simulink model "RxCAN2"  (R2014a)
settings: Solver=ode45  StartTime=0.0  StopTime=10.0  RelTol=1e-3
libraries: simulink x16
settings Model: Creator=10226  LastModifiedBy=10226

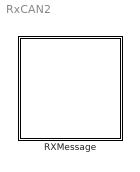
== system RxCAN2 ==
  RXMessage : Subsystem

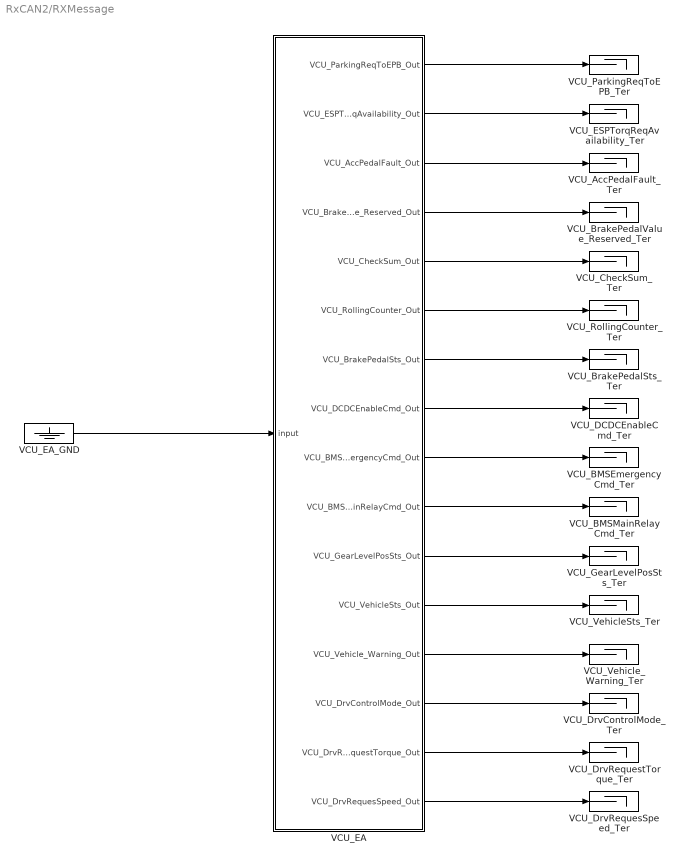
== system RxCAN2/RXMessage ==
  VCU_AccPedalFault_Ter : Terminator
  VCU_BMSEmergencyCmd_Ter : Terminator
  VCU_BMSMainRelayCmd_Ter : Terminator
  VCU_BrakePedalSts_Ter : Terminator
  VCU_BrakePedalValue_Reserved_Ter : Terminator
  VCU_CheckSum_Ter : Terminator
  VCU_DCDCEnableCmd_Ter : Terminator
  VCU_DrvControlMode_Ter : Terminator
  VCU_DrvRequesSpeed_Ter : Terminator
  VCU_DrvRequestTorque_Ter : Terminator
  VCU_EA : Subsystem
  VCU_EA_GND : Ground
  VCU_ESPTorqReqAvailability_Ter : Terminator
  VCU_GearLevelPosSts_Ter : Terminator
  VCU_ParkingReqToEPB_Ter : Terminator
  VCU_RollingCounter_Ter : Terminator
  VCU_VehicleSts_Ter : Terminator
  VCU_Vehicle_Warning_Ter : Terminator
  wires:
  VCU_EA/1(VCU_ParkingReqToEPB_Out) -> VCU_ParkingReqToEPB_Ter/1
  VCU_EA/2(VCU_ESPTorqReqAvailability_Out) -> VCU_ESPTorqReqAvailability_Ter/1
  VCU_EA/3(VCU_AccPedalFault_Out) -> VCU_AccPedalFault_Ter/1
  VCU_EA/4(VCU_BrakePedalValue_Reserved_Out) -> VCU_BrakePedalValue_Reserved_Ter/1
  VCU_EA/5(VCU_CheckSum_Out) -> VCU_CheckSum_Ter/1
  VCU_EA/6(VCU_RollingCounter_Out) -> VCU_RollingCounter_Ter/1
  VCU_EA/7(VCU_BrakePedalSts_Out) -> VCU_BrakePedalSts_Ter/1
  VCU_EA/8(VCU_DCDCEnableCmd_Out) -> VCU_DCDCEnableCmd_Ter/1
  VCU_EA/9(VCU_BMSEmergencyCmd_Out) -> VCU_BMSEmergencyCmd_Ter/1
  VCU_EA/10(VCU_BMSMainRelayCmd_Out) -> VCU_BMSMainRelayCmd_Ter/1
  VCU_EA/11(VCU_GearLevelPosSts_Out) -> VCU_GearLevelPosSts_Ter/1
  VCU_EA/12(VCU_VehicleSts_Out) -> VCU_VehicleSts_Ter/1
  VCU_EA/13(VCU_Vehicle_Warning_Out) -> VCU_Vehicle_Warning_Ter/1
  VCU_EA/14(VCU_DrvControlMode_Out) -> VCU_DrvControlMode_Ter/1
  VCU_EA/15(VCU_DrvRequestTorque_Out) -> VCU_DrvRequestTorque_Ter/1
  VCU_EA/16(VCU_DrvRequesSpeed_Out) -> VCU_DrvRequesSpeed_Ter/1
  VCU_EA_GND/1 -> VCU_EA/1(input)

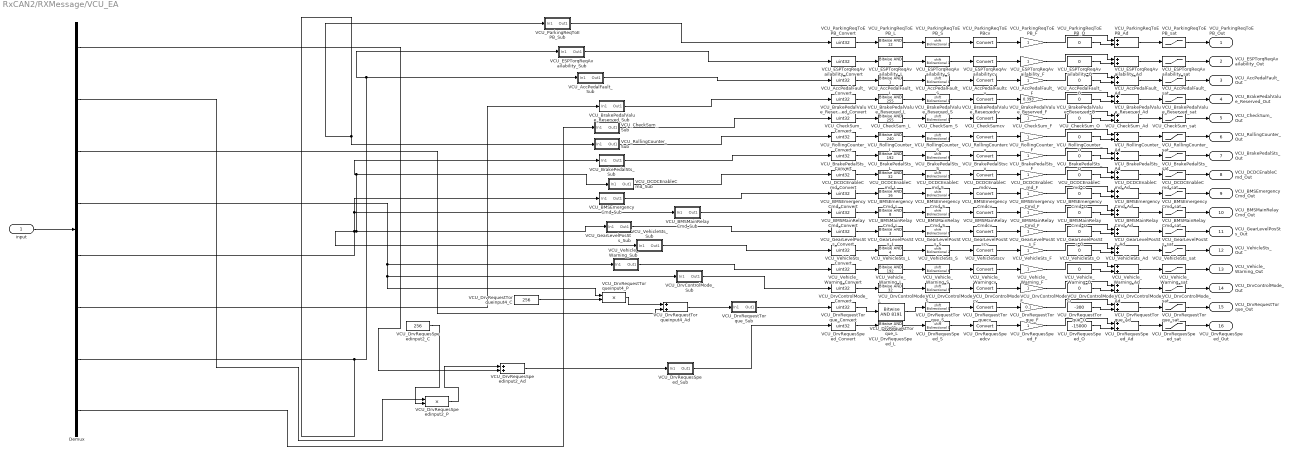
== system RxCAN2/RXMessage/VCU_EA ==
  input : Inport
  Demux : Demux  Outputs=8
  VCU_AccPedalFault_Ad : Sum
  VCU_AccPedalFault_Convert : DataTypeConversion  OutDataTypeStr=uint32
  VCU_AccPedalFault_F : Gain
  VCU_AccPedalFault_L : simulink/Logic and Bit Operations/Bitwise Operator  logicop=AND  UseBitMask=on  BitMask=1  BitMaskRealWorld=Stored Integer
  VCU_AccPedalFault_O : Constant  Value=0  OutDataTypeStr=single
  VCU_AccPedalFault_S : ArithShift
  VCU_AccPedalFault_Sub : Subsystem
  VCU_AccPedalFault_sat : Saturate  UpperLimit=1  LowerLimit=0
  VCU_AccPedalFaultcv : DataTypeConversion
  VCU_BMSEmergencyCmd_Ad : Sum
  VCU_BMSEmergencyCmd_Convert : DataTypeConversion  OutDataTypeStr=uint32
  VCU_BMSEmergencyCmd_F : Gain
  VCU_BMSEmergencyCmd_L : simulink/Logic and Bit Operations/Bitwise Operator  logicop=AND  UseBitMask=on  BitMask=16  BitMaskRealWorld=Stored Integer
  VCU_BMSEmergencyCmd_O : Constant  Value=0  OutDataTypeStr=single
  VCU_BMSEmergencyCmd_S : ArithShift  BitShiftNumber=4
  VCU_BMSEmergencyCmd_Sub : Subsystem
  VCU_BMSEmergencyCmd_sat : Saturate  UpperLimit=1  LowerLimit=0
  VCU_BMSEmergencyCmdcv : DataTypeConversion
  VCU_BMSMainRelayCmd_Ad : Sum
  VCU_BMSMainRelayCmd_Convert : DataTypeConversion  OutDataTypeStr=uint32
  VCU_BMSMainRelayCmd_F : Gain
  VCU_BMSMainRelayCmd_L : simulink/Logic and Bit Operations/Bitwise Operator  logicop=AND  UseBitMask=on  BitMask=8  BitMaskRealWorld=Stored Integer
  VCU_BMSMainRelayCmd_O : Constant  Value=0  OutDataTypeStr=single
  VCU_BMSMainRelayCmd_S : ArithShift  BitShiftNumber=3
  VCU_BMSMainRelayCmd_Sub : Subsystem
  VCU_BMSMainRelayCmd_sat : Saturate  UpperLimit=1  LowerLimit=0
  VCU_BMSMainRelayCmdcv : DataTypeConversion
  VCU_BrakePedalSts_Ad : Sum
  VCU_BrakePedalSts_Convert : DataTypeConversion  OutDataTypeStr=uint32
  VCU_BrakePedalSts_F : Gain
  VCU_BrakePedalSts_L : simulink/Logic and Bit Operations/Bitwise Operator  logicop=AND  UseBitMask=on  BitMask=192  BitMaskRealWorld=Stored Integer
  VCU_BrakePedalSts_O : Constant  Value=0  OutDataTypeStr=single
  VCU_BrakePedalSts_S : ArithShift  BitShiftNumber=6
  VCU_BrakePedalSts_Sub : Subsystem
  VCU_BrakePedalSts_sat : Saturate  UpperLimit=3  LowerLimit=0
  VCU_BrakePedalStscv : DataTypeConversion
  VCU_BrakePedalValue_Reserved_Ad : Sum
  VCU_BrakePedalValue_Reserved_Convert : DataTypeConversion  OutDataTypeStr=uint32
  VCU_BrakePedalValue_Reserved_F : Gain  Gain=0.393
  VCU_BrakePedalValue_Reserved_L : simulink/Logic and Bit Operations/Bitwise Operator  logicop=AND  UseBitMask=on  BitMask=255  BitMaskRealWorld=Stored Integer
  VCU_BrakePedalValue_Reserved_O : Constant  Value=0  OutDataTypeStr=single
  VCU_BrakePedalValue_Reserved_S : ArithShift
  VCU_BrakePedalValue_Reserved_Sub : Subsystem
  VCU_BrakePedalValue_Reserved_sat : Saturate  UpperLimit=100  LowerLimit=0
  VCU_BrakePedalValue_Reservedcv : DataTypeConversion
  VCU_CheckSum_Ad : Sum
  VCU_CheckSum_Convert : DataTypeConversion  OutDataTypeStr=uint32
  VCU_CheckSum_F : Gain
  VCU_CheckSum_L : simulink/Logic and Bit Operations/Bitwise Operator  logicop=AND  UseBitMask=on  BitMask=255  BitMaskRealWorld=Stored Integer
  VCU_CheckSum_O : Constant  Value=0  OutDataTypeStr=single
  VCU_CheckSum_S : ArithShift
  VCU_CheckSum_Sub : Subsystem
  VCU_CheckSum_sat : Saturate  UpperLimit=255  LowerLimit=0
  VCU_CheckSumcv : DataTypeConversion
  VCU_DCDCEnableCmd_Ad : Sum
  VCU_DCDCEnableCmd_Convert : DataTypeConversion  OutDataTypeStr=uint32
  VCU_DCDCEnableCmd_F : Gain
  VCU_DCDCEnableCmd_L : simulink/Logic and Bit Operations/Bitwise Operator  logicop=AND  UseBitMask=on  BitMask=32  BitMaskRealWorld=Stored Integer
  VCU_DCDCEnableCmd_O : Constant  Value=0  OutDataTypeStr=single
  VCU_DCDCEnableCmd_S : ArithShift  BitShiftNumber=5
  VCU_DCDCEnableCmd_Sub : Subsystem
  VCU_DCDCEnableCmd_sat : Saturate  UpperLimit=1  LowerLimit=0
  VCU_DCDCEnableCmdcv : DataTypeConversion
  VCU_DrvControlMode_Ad : Sum
  VCU_DrvControlMode_Convert : DataTypeConversion  OutDataTypeStr=uint32
  VCU_DrvControlMode_F : Gain
  VCU_DrvControlMode_L : simulink/Logic and Bit Operations/Bitwise Operator  logicop=AND  UseBitMask=on  BitMask=32  BitMaskRealWorld=Stored Integer
  VCU_DrvControlMode_O : Constant  Value=0  OutDataTypeStr=single
  VCU_DrvControlMode_S : ArithShift  BitShiftNumber=5
  VCU_DrvControlMode_Sub : Subsystem
  VCU_DrvControlMode_sat : Saturate  UpperLimit=1  LowerLimit=0
  VCU_DrvControlModecv : DataTypeConversion
  VCU_DrvRequesSpeed_Ad : Sum
  VCU_DrvRequesSpeed_Convert : DataTypeConversion  OutDataTypeStr=uint32
  VCU_DrvRequesSpeed_F : Gain
  VCU_DrvRequesSpeed_L : simulink/Logic and Bit Operations/Bitwise Operator  logicop=AND  UseBitMask=on  BitMask=65535  BitMaskRealWorld=Stored Integer
  VCU_DrvRequesSpeed_O : Constant  Value=-15000  OutDataTypeStr=single
  VCU_DrvRequesSpeed_S : ArithShift
  VCU_DrvRequesSpeed_Sub : Subsystem
  VCU_DrvRequesSpeed_sat : Saturate  UpperLimit=15000  LowerLimit=-15000
  VCU_DrvRequesSpeedcv : DataTypeConversion
  VCU_DrvRequesSpeedinput2_Ad : Sum
  VCU_DrvRequesSpeedinput2_C : Constant  Value=256
  VCU_DrvRequesSpeedinput2_P : Product
  VCU_DrvRequestTorque_Ad : Sum
  VCU_DrvRequestTorque_Convert : DataTypeConversion  OutDataTypeStr=uint32
  VCU_DrvRequestTorque_F : Gain  Gain=0.1
  VCU_DrvRequestTorque_L : simulink/Logic and Bit Operations/Bitwise Operator  logicop=AND  UseBitMask=on  BitMask=8191  BitMaskRealWorld=Stored Integer
  VCU_DrvRequestTorque_O : Constant  Value=-300  OutDataTypeStr=single
  VCU_DrvRequestTorque_S : ArithShift
  VCU_DrvRequestTorque_Sub : Subsystem
  VCU_DrvRequestTorque_sat : Saturate  UpperLimit=300  LowerLimit=-300
  VCU_DrvRequestTorquecv : DataTypeConversion
  VCU_DrvRequestTorqueinput4_Ad : Sum
  VCU_DrvRequestTorqueinput4_C : Constant  Value=256
  VCU_DrvRequestTorqueinput4_P : Product
  VCU_ESPTorqReqAvailability_Ad : Sum
  VCU_ESPTorqReqAvailability_Convert : DataTypeConversion  OutDataTypeStr=uint32
  VCU_ESPTorqReqAvailability_F : Gain
  VCU_ESPTorqReqAvailability_L : simulink/Logic and Bit Operations/Bitwise Operator  logicop=AND  UseBitMask=on  BitMask=2  BitMaskRealWorld=Stored Integer
  VCU_ESPTorqReqAvailability_O : Constant  Value=0  OutDataTypeStr=single
  VCU_ESPTorqReqAvailability_S : ArithShift  BitShiftNumber=1
  VCU_ESPTorqReqAvailability_Sub : Subsystem
  VCU_ESPTorqReqAvailability_sat : Saturate  UpperLimit=1  LowerLimit=0
  VCU_ESPTorqReqAvailabilitycv : DataTypeConversion
  VCU_GearLevelPosSts_Ad : Sum
  VCU_GearLevelPosSts_Convert : DataTypeConversion  OutDataTypeStr=uint32
  VCU_GearLevelPosSts_F : Gain
  VCU_GearLevelPosSts_L : simulink/Logic and Bit Operations/Bitwise Operator  logicop=AND  UseBitMask=on  BitMask=3  BitMaskRealWorld=Stored Integer
  VCU_GearLevelPosSts_O : Constant  Value=0  OutDataTypeStr=single
  VCU_GearLevelPosSts_S : ArithShift
  VCU_GearLevelPosSts_Sub : Subsystem
  VCU_GearLevelPosSts_sat : Saturate  UpperLimit=3  LowerLimit=0
  VCU_GearLevelPosStscv : DataTypeConversion
  VCU_ParkingReqToEPB_Ad : Sum
  VCU_ParkingReqToEPB_Convert : DataTypeConversion  OutDataTypeStr=uint32
  VCU_ParkingReqToEPB_F : Gain
  VCU_ParkingReqToEPB_L : simulink/Logic and Bit Operations/Bitwise Operator  logicop=AND  UseBitMask=on  BitMask=12  BitMaskRealWorld=Stored Integer
  VCU_ParkingReqToEPB_O : Constant  Value=0  OutDataTypeStr=single
  VCU_ParkingReqToEPB_S : ArithShift  BitShiftNumber=2
  VCU_ParkingReqToEPB_Sub : Subsystem
  VCU_ParkingReqToEPB_sat : Saturate  UpperLimit=3  LowerLimit=0
  VCU_ParkingReqToEPBcv : DataTypeConversion
  VCU_RollingCounter_Ad : Sum
  VCU_RollingCounter_Convert : DataTypeConversion  OutDataTypeStr=uint32
  VCU_RollingCounter_F : Gain
  VCU_RollingCounter_L : simulink/Logic and Bit Operations/Bitwise Operator  logicop=AND  UseBitMask=on  BitMask=240  BitMaskRealWorld=Stored Integer
  VCU_RollingCounter_O : Constant  Value=0  OutDataTypeStr=single
  VCU_RollingCounter_S : ArithShift  BitShiftNumber=4
  VCU_RollingCounter_Sub : Subsystem
  VCU_RollingCounter_sat : Saturate  UpperLimit=15  LowerLimit=0
  VCU_RollingCountercv : DataTypeConversion
  VCU_VehicleSts_Ad : Sum
  VCU_VehicleSts_Convert : DataTypeConversion  OutDataTypeStr=uint32
  VCU_VehicleSts_F : Gain
  VCU_VehicleSts_L : simulink/Logic and Bit Operations/Bitwise Operator  logicop=AND  UseBitMask=on  BitMask=4  BitMaskRealWorld=Stored Integer
  VCU_VehicleSts_O : Constant  Value=0  OutDataTypeStr=single
  VCU_VehicleSts_S : ArithShift  BitShiftNumber=2
  VCU_VehicleSts_Sub : Subsystem
  VCU_VehicleSts_sat : Saturate  UpperLimit=1  LowerLimit=0
  VCU_VehicleStscv : DataTypeConversion
  VCU_Vehicle_Warning_Ad : Sum
  VCU_Vehicle_Warning_Convert : DataTypeConversion  OutDataTypeStr=uint32
  VCU_Vehicle_Warning_F : Gain
  VCU_Vehicle_Warning_L : simulink/Logic and Bit Operations/Bitwise Operator  logicop=AND  UseBitMask=on  BitMask=192  BitMaskRealWorld=Stored Integer
  VCU_Vehicle_Warning_O : Constant  Value=0  OutDataTypeStr=single
  VCU_Vehicle_Warning_S : ArithShift  BitShiftNumber=6
  VCU_Vehicle_Warning_Sub : Subsystem
  VCU_Vehicle_Warning_sat : Saturate  UpperLimit=3  LowerLimit=0
  VCU_Vehicle_Warningcv : DataTypeConversion
  VCU_ParkingReqToEPB_Out : Outport
  VCU_ESPTorqReqAvailability_Out : Outport  Port=2
  VCU_AccPedalFault_Out : Outport  Port=3
  VCU_BrakePedalValue_Reserved_Out : Outport  Port=4
  VCU_CheckSum_Out : Outport  Port=5
  VCU_RollingCounter_Out : Outport  Port=6
  VCU_BrakePedalSts_Out : Outport  Port=7
  VCU_DCDCEnableCmd_Out : Outport  Port=8
  VCU_BMSEmergencyCmd_Out : Outport  Port=9
  VCU_BMSMainRelayCmd_Out : Outport  Port=10
  VCU_GearLevelPosSts_Out : Outport  Port=11
  VCU_VehicleSts_Out : Outport  Port=12
  VCU_Vehicle_Warning_Out : Outport  Port=13
  VCU_DrvControlMode_Out : Outport  Port=14
  VCU_DrvRequestTorque_Out : Outport  Port=15
  VCU_DrvRequesSpeed_Out : Outport  Port=16
  wires:
  VCU_ParkingReqToEPB_F/1 -> VCU_ParkingReqToEPB_Ad/1
  VCU_ParkingReqToEPB_O/1 -> VCU_ParkingReqToEPB_Ad/2
  VCU_ParkingReqToEPB_Ad/1 -> VCU_ParkingReqToEPB_sat/1
  VCU_ParkingReqToEPB_sat/1 -> VCU_ParkingReqToEPB_Out/1
  Demux/7 -> VCU_ESPTorqReqAvailability_Sub/1(In1), VCU_AccPedalFault_Sub/1(In1), VCU_RollingCounter_Sub/1(In1), VCU_ParkingReqToEPB_Sub/1(In1)
  VCU_ParkingReqToEPB_Sub/1(Out1) -> VCU_ParkingReqToEPB_Convert/1
  VCU_ParkingReqToEPB_Convert/1 -> VCU_ParkingReqToEPB_L/1
  VCU_ParkingReqToEPB_L/1 -> VCU_ParkingReqToEPB_S/1
  VCU_ParkingReqToEPB_S/1 -> VCU_ParkingReqToEPBcv/1
  VCU_ParkingReqToEPBcv/1 -> VCU_ParkingReqToEPB_F/1
  VCU_ESPTorqReqAvailability_F/1 -> VCU_ESPTorqReqAvailability_Ad/1
  VCU_ESPTorqReqAvailability_O/1 -> VCU_ESPTorqReqAvailability_Ad/2
  VCU_ESPTorqReqAvailability_Ad/1 -> VCU_ESPTorqReqAvailability_sat/1
  VCU_ESPTorqReqAvailability_sat/1 -> VCU_ESPTorqReqAvailability_Out/1
  VCU_ESPTorqReqAvailability_Sub/1(Out1) -> VCU_ESPTorqReqAvailability_Convert/1
  VCU_ESPTorqReqAvailability_Convert/1 -> VCU_ESPTorqReqAvailability_L/1
  VCU_ESPTorqReqAvailability_L/1 -> VCU_ESPTorqReqAvailability_S/1
  VCU_ESPTorqReqAvailability_S/1 -> VCU_ESPTorqReqAvailabilitycv/1
  VCU_ESPTorqReqAvailabilitycv/1 -> VCU_ESPTorqReqAvailability_F/1
  VCU_AccPedalFault_F/1 -> VCU_AccPedalFault_Ad/1
  VCU_AccPedalFault_O/1 -> VCU_AccPedalFault_Ad/2
  VCU_AccPedalFault_Ad/1 -> VCU_AccPedalFault_sat/1
  VCU_AccPedalFault_sat/1 -> VCU_AccPedalFault_Out/1
  VCU_AccPedalFault_Sub/1(Out1) -> VCU_AccPedalFault_Convert/1
  VCU_AccPedalFault_Convert/1 -> VCU_AccPedalFault_L/1
  VCU_AccPedalFault_L/1 -> VCU_AccPedalFault_S/1
  VCU_AccPedalFault_S/1 -> VCU_AccPedalFaultcv/1
  VCU_AccPedalFaultcv/1 -> VCU_AccPedalFault_F/1
  VCU_BrakePedalValue_Reserved_F/1 -> VCU_BrakePedalValue_Reserved_Ad/1
  VCU_BrakePedalValue_Reserved_O/1 -> VCU_BrakePedalValue_Reserved_Ad/2
  VCU_BrakePedalValue_Reserved_Ad/1 -> VCU_BrakePedalValue_Reserved_sat/1
  VCU_BrakePedalValue_Reserved_sat/1 -> VCU_BrakePedalValue_Reserved_Out/1
  Demux/6 -> VCU_BrakePedalValue_Reserved_Sub/1(In1)
  VCU_BrakePedalValue_Reserved_Sub/1(Out1) -> VCU_BrakePedalValue_Reserved_Convert/1
  VCU_BrakePedalValue_Reserved_Convert/1 -> VCU_BrakePedalValue_Reserved_L/1
  VCU_BrakePedalValue_Reserved_L/1 -> VCU_BrakePedalValue_Reserved_S/1
  VCU_BrakePedalValue_Reserved_S/1 -> VCU_BrakePedalValue_Reservedcv/1
  VCU_BrakePedalValue_Reservedcv/1 -> VCU_BrakePedalValue_Reserved_F/1
  VCU_CheckSum_F/1 -> VCU_CheckSum_Ad/1
  VCU_CheckSum_O/1 -> VCU_CheckSum_Ad/2
  VCU_CheckSum_Ad/1 -> VCU_CheckSum_sat/1
  VCU_CheckSum_sat/1 -> VCU_CheckSum_Out/1
  Demux/8 -> VCU_CheckSum_Sub/1(In1)
  VCU_CheckSum_Sub/1(Out1) -> VCU_CheckSum_Convert/1
  VCU_CheckSum_Convert/1 -> VCU_CheckSum_L/1
  VCU_CheckSum_L/1 -> VCU_CheckSum_S/1
  VCU_CheckSum_S/1 -> VCU_CheckSumcv/1
  VCU_CheckSumcv/1 -> VCU_CheckSum_F/1
  VCU_RollingCounter_F/1 -> VCU_RollingCounter_Ad/1
  VCU_RollingCounter_O/1 -> VCU_RollingCounter_Ad/2
  VCU_RollingCounter_Ad/1 -> VCU_RollingCounter_sat/1
  VCU_RollingCounter_sat/1 -> VCU_RollingCounter_Out/1
  VCU_RollingCounter_Sub/1(Out1) -> VCU_RollingCounter_Convert/1
  VCU_RollingCounter_Convert/1 -> VCU_RollingCounter_L/1
  VCU_RollingCounter_L/1 -> VCU_RollingCounter_S/1
  VCU_RollingCounter_S/1 -> VCU_RollingCountercv/1
  VCU_RollingCountercv/1 -> VCU_RollingCounter_F/1
  VCU_BrakePedalSts_F/1 -> VCU_BrakePedalSts_Ad/1
  VCU_BrakePedalSts_O/1 -> VCU_BrakePedalSts_Ad/2
  VCU_BrakePedalSts_Ad/1 -> VCU_BrakePedalSts_sat/1
  VCU_BrakePedalSts_sat/1 -> VCU_BrakePedalSts_Out/1
  Demux/5 -> VCU_GearLevelPosSts_Sub/1(In1), VCU_BrakePedalSts_Sub/1(In1), VCU_DCDCEnableCmd_Sub/1(In1), VCU_VehicleSts_Sub/1(In1), VCU_BMSEmergencyCmd_Sub/1(In1), VCU_BMSMainRelayCmd_Sub/1(In1)
  VCU_BrakePedalSts_Sub/1(Out1) -> VCU_BrakePedalSts_Convert/1
  VCU_BrakePedalSts_Convert/1 -> VCU_BrakePedalSts_L/1
  VCU_BrakePedalSts_L/1 -> VCU_BrakePedalSts_S/1
  VCU_BrakePedalSts_S/1 -> VCU_BrakePedalStscv/1
  VCU_BrakePedalStscv/1 -> VCU_BrakePedalSts_F/1
  VCU_DCDCEnableCmd_F/1 -> VCU_DCDCEnableCmd_Ad/1
  VCU_DCDCEnableCmd_O/1 -> VCU_DCDCEnableCmd_Ad/2
  VCU_DCDCEnableCmd_Ad/1 -> VCU_DCDCEnableCmd_sat/1
  VCU_DCDCEnableCmd_sat/1 -> VCU_DCDCEnableCmd_Out/1
  VCU_DCDCEnableCmd_Sub/1(Out1) -> VCU_DCDCEnableCmd_Convert/1
  VCU_DCDCEnableCmd_Convert/1 -> VCU_DCDCEnableCmd_L/1
  VCU_DCDCEnableCmd_L/1 -> VCU_DCDCEnableCmd_S/1
  VCU_DCDCEnableCmd_S/1 -> VCU_DCDCEnableCmdcv/1
  VCU_DCDCEnableCmdcv/1 -> VCU_DCDCEnableCmd_F/1
  VCU_BMSEmergencyCmd_F/1 -> VCU_BMSEmergencyCmd_Ad/1
  VCU_BMSEmergencyCmd_O/1 -> VCU_BMSEmergencyCmd_Ad/2
  VCU_BMSEmergencyCmd_Ad/1 -> VCU_BMSEmergencyCmd_sat/1
  VCU_BMSEmergencyCmd_sat/1 -> VCU_BMSEmergencyCmd_Out/1
  VCU_BMSEmergencyCmd_Sub/1(Out1) -> VCU_BMSEmergencyCmd_Convert/1
  VCU_BMSEmergencyCmd_Convert/1 -> VCU_BMSEmergencyCmd_L/1
  VCU_BMSEmergencyCmd_L/1 -> VCU_BMSEmergencyCmd_S/1
  VCU_BMSEmergencyCmd_S/1 -> VCU_BMSEmergencyCmdcv/1
  VCU_BMSEmergencyCmdcv/1 -> VCU_BMSEmergencyCmd_F/1
  VCU_BMSMainRelayCmd_F/1 -> VCU_BMSMainRelayCmd_Ad/1
  VCU_BMSMainRelayCmd_O/1 -> VCU_BMSMainRelayCmd_Ad/2
  VCU_BMSMainRelayCmd_Ad/1 -> VCU_BMSMainRelayCmd_sat/1
  VCU_BMSMainRelayCmd_sat/1 -> VCU_BMSMainRelayCmd_Out/1
  VCU_BMSMainRelayCmd_Sub/1(Out1) -> VCU_BMSMainRelayCmd_Convert/1
  VCU_BMSMainRelayCmd_Convert/1 -> VCU_BMSMainRelayCmd_L/1
  VCU_BMSMainRelayCmd_L/1 -> VCU_BMSMainRelayCmd_S/1
  VCU_BMSMainRelayCmd_S/1 -> VCU_BMSMainRelayCmdcv/1
  VCU_BMSMainRelayCmdcv/1 -> VCU_BMSMainRelayCmd_F/1
  VCU_GearLevelPosSts_F/1 -> VCU_GearLevelPosSts_Ad/1
  VCU_GearLevelPosSts_O/1 -> VCU_GearLevelPosSts_Ad/2
  VCU_GearLevelPosSts_Ad/1 -> VCU_GearLevelPosSts_sat/1
  VCU_GearLevelPosSts_sat/1 -> VCU_GearLevelPosSts_Out/1
  VCU_GearLevelPosSts_Sub/1(Out1) -> VCU_GearLevelPosSts_Convert/1
  VCU_GearLevelPosSts_Convert/1 -> VCU_GearLevelPosSts_L/1
  VCU_GearLevelPosSts_L/1 -> VCU_GearLevelPosSts_S/1
  VCU_GearLevelPosSts_S/1 -> VCU_GearLevelPosStscv/1
  VCU_GearLevelPosStscv/1 -> VCU_GearLevelPosSts_F/1
  VCU_VehicleSts_F/1 -> VCU_VehicleSts_Ad/1
  VCU_VehicleSts_O/1 -> VCU_VehicleSts_Ad/2
  VCU_VehicleSts_Ad/1 -> VCU_VehicleSts_sat/1
  VCU_VehicleSts_sat/1 -> VCU_VehicleSts_Out/1
  VCU_VehicleSts_Sub/1(Out1) -> VCU_VehicleSts_Convert/1
  VCU_VehicleSts_Convert/1 -> VCU_VehicleSts_L/1
  VCU_VehicleSts_L/1 -> VCU_VehicleSts_S/1
  VCU_VehicleSts_S/1 -> VCU_VehicleStscv/1
  VCU_VehicleStscv/1 -> VCU_VehicleSts_F/1
  VCU_Vehicle_Warning_F/1 -> VCU_Vehicle_Warning_Ad/1
  VCU_Vehicle_Warning_O/1 -> VCU_Vehicle_Warning_Ad/2
  VCU_Vehicle_Warning_Ad/1 -> VCU_Vehicle_Warning_sat/1
  VCU_Vehicle_Warning_sat/1 -> VCU_Vehicle_Warning_Out/1
  Demux/4 -> VCU_DrvRequestTorqueinput4_P/1, VCU_DrvControlMode_Sub/1(In1), VCU_Vehicle_Warning_Sub/1(In1)
  VCU_Vehicle_Warning_Sub/1(Out1) -> VCU_Vehicle_Warning_Convert/1
  VCU_Vehicle_Warning_Convert/1 -> VCU_Vehicle_Warning_L/1
  VCU_Vehicle_Warning_L/1 -> VCU_Vehicle_Warning_S/1
  VCU_Vehicle_Warning_S/1 -> VCU_Vehicle_Warningcv/1
  VCU_Vehicle_Warningcv/1 -> VCU_Vehicle_Warning_F/1
  VCU_DrvControlMode_F/1 -> VCU_DrvControlMode_Ad/1
  VCU_DrvControlMode_O/1 -> VCU_DrvControlMode_Ad/2
  VCU_DrvControlMode_Ad/1 -> VCU_DrvControlMode_sat/1
  VCU_DrvControlMode_sat/1 -> VCU_DrvControlMode_Out/1
  VCU_DrvControlMode_Sub/1(Out1) -> VCU_DrvControlMode_Convert/1
  VCU_DrvControlMode_Convert/1 -> VCU_DrvControlMode_L/1
  VCU_DrvControlMode_L/1 -> VCU_DrvControlMode_S/1
  VCU_DrvControlMode_S/1 -> VCU_DrvControlModecv/1
  VCU_DrvControlModecv/1 -> VCU_DrvControlMode_F/1
  VCU_DrvRequestTorque_F/1 -> VCU_DrvRequestTorque_Ad/1
  VCU_DrvRequestTorque_O/1 -> VCU_DrvRequestTorque_Ad/2
  VCU_DrvRequestTorque_Ad/1 -> VCU_DrvRequestTorque_sat/1
  VCU_DrvRequestTorque_sat/1 -> VCU_DrvRequestTorque_Out/1
  VCU_DrvRequestTorqueinput4_C/1 -> VCU_DrvRequestTorqueinput4_P/2
  VCU_DrvRequestTorqueinput4_P/1 -> VCU_DrvRequestTorqueinput4_Ad/1
  Demux/3 -> VCU_DrvRequestTorqueinput4_Ad/2
  VCU_DrvRequestTorqueinput4_Ad/1 -> VCU_DrvRequestTorque_Sub/1(In1)
  VCU_DrvRequestTorque_Sub/1(Out1) -> VCU_DrvRequestTorque_Convert/1
  VCU_DrvRequestTorque_Convert/1 -> VCU_DrvRequestTorque_L/1
  VCU_DrvRequestTorque_L/1 -> VCU_DrvRequestTorque_S/1
  VCU_DrvRequestTorque_S/1 -> VCU_DrvRequestTorquecv/1
  VCU_DrvRequestTorquecv/1 -> VCU_DrvRequestTorque_F/1
  VCU_DrvRequesSpeed_F/1 -> VCU_DrvRequesSpeed_Ad/1
  VCU_DrvRequesSpeed_O/1 -> VCU_DrvRequesSpeed_Ad/2
  VCU_DrvRequesSpeed_Ad/1 -> VCU_DrvRequesSpeed_sat/1
  VCU_DrvRequesSpeed_sat/1 -> VCU_DrvRequesSpeed_Out/1
  Demux/2 -> VCU_DrvRequesSpeedinput2_P/1
  VCU_DrvRequesSpeedinput2_C/1 -> VCU_DrvRequesSpeedinput2_P/2
  VCU_DrvRequesSpeedinput2_P/1 -> VCU_DrvRequesSpeedinput2_Ad/1
  Demux/1 -> VCU_DrvRequesSpeedinput2_Ad/2
  VCU_DrvRequesSpeedinput2_Ad/1 -> VCU_DrvRequesSpeed_Sub/1(In1)
  VCU_DrvRequesSpeed_Sub/1(Out1) -> VCU_DrvRequesSpeed_Convert/1
  VCU_DrvRequesSpeed_Convert/1 -> VCU_DrvRequesSpeed_L/1
  VCU_DrvRequesSpeed_L/1 -> VCU_DrvRequesSpeed_S/1
  VCU_DrvRequesSpeed_S/1 -> VCU_DrvRequesSpeedcv/1
  VCU_DrvRequesSpeedcv/1 -> VCU_DrvRequesSpeed_F/1
  input/1 -> Demux/1

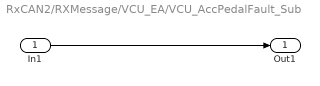
== system RxCAN2/RXMessage/VCU_EA/VCU_AccPedalFault_Sub ==
  In1 : Inport
  Out1 : Outport
  wires:
  In1/1 -> Out1/1

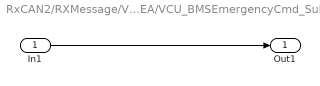
== system RxCAN2/RXMessage/VCU_EA/VCU_BMSEmergencyCmd_Sub ==
  In1 : Inport
  Out1 : Outport
  wires:
  In1/1 -> Out1/1

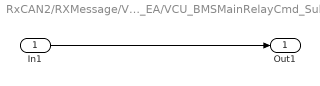
== system RxCAN2/RXMessage/VCU_EA/VCU_BMSMainRelayCmd_Sub ==
  In1 : Inport
  Out1 : Outport
  wires:
  In1/1 -> Out1/1

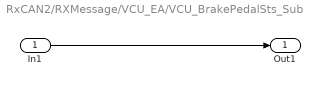
== system RxCAN2/RXMessage/VCU_EA/VCU_BrakePedalSts_Sub ==
  In1 : Inport
  Out1 : Outport
  wires:
  In1/1 -> Out1/1

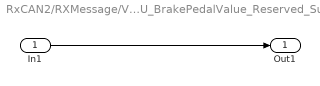
== system RxCAN2/RXMessage/VCU_EA/VCU_BrakePedalValue_Reserved_Sub ==
  In1 : Inport
  Out1 : Outport
  wires:
  In1/1 -> Out1/1

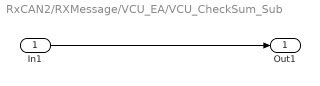
== system RxCAN2/RXMessage/VCU_EA/VCU_CheckSum_Sub ==
  In1 : Inport
  Out1 : Outport
  wires:
  In1/1 -> Out1/1

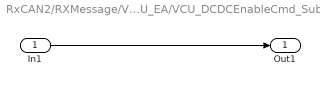
== system RxCAN2/RXMessage/VCU_EA/VCU_DCDCEnableCmd_Sub ==
  In1 : Inport
  Out1 : Outport
  wires:
  In1/1 -> Out1/1

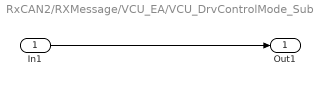
== system RxCAN2/RXMessage/VCU_EA/VCU_DrvControlMode_Sub ==
  In1 : Inport
  Out1 : Outport
  wires:
  In1/1 -> Out1/1

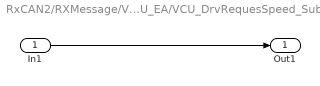
== system RxCAN2/RXMessage/VCU_EA/VCU_DrvRequesSpeed_Sub ==
  In1 : Inport
  Out1 : Outport
  wires:
  In1/1 -> Out1/1

== system RxCAN2/RXMessage/VCU_EA/VCU_DrvRequestTorque_Sub ==
  In1 : Inport
  Out1 : Outport
  wires:
  In1/1 -> Out1/1

== system RxCAN2/RXMessage/VCU_EA/VCU_ESPTorqReqAvailability_Sub ==
  In1 : Inport
  Out1 : Outport
  wires:
  In1/1 -> Out1/1

== system RxCAN2/RXMessage/VCU_EA/VCU_GearLevelPosSts_Sub ==
  In1 : Inport
  Out1 : Outport
  wires:
  In1/1 -> Out1/1

== system RxCAN2/RXMessage/VCU_EA/VCU_ParkingReqToEPB_Sub ==
  In1 : Inport
  Out1 : Outport
  wires:
  In1/1 -> Out1/1

== system RxCAN2/RXMessage/VCU_EA/VCU_RollingCounter_Sub ==
  In1 : Inport
  Out1 : Outport
  wires:
  In1/1 -> Out1/1

== system RxCAN2/RXMessage/VCU_EA/VCU_VehicleSts_Sub ==
  In1 : Inport
  Out1 : Outport
  wires:
  In1/1 -> Out1/1

== system RxCAN2/RXMessage/VCU_EA/VCU_Vehicle_Warning_Sub ==
  In1 : Inport
  Out1 : Outport
  wires:
  In1/1 -> Out1/1
